simulink model "offGrid_Inverter"  (R2022b)
settings: Solver=FixedStepDiscrete  StartTime=0.0  StopTime=2  FixedStep=1e-6  RelTol=1e-3
libraries: spsSeriesRLCBranchLib x11, spsCurrentMeasurementLib x7, spsMosfetLib x6, slpidlib x5, spsRMSLib x4, simulink x4, spsFourierLib x2, spsTriangleGeneratorLib x2, spsVoltageMeasurementLib x2, spsBreakerLib x1, spsDCVoltageSourceLib x1, spspowerguiLib x1
(part 1 of 2)
settings Model: Creator=XIAO  LastModifiedBy=XIAO
settings SolverCC: AutoInsertRateTranBlk=on
settings DataIOCC: ReturnWorkspaceOutputs=off

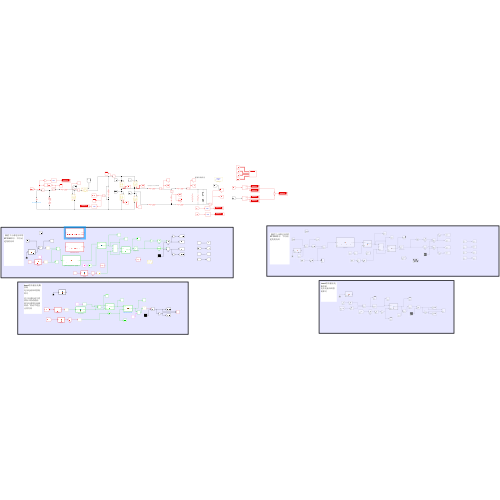
[thumbnail: Simulink's stored preview of the top-level diagram]
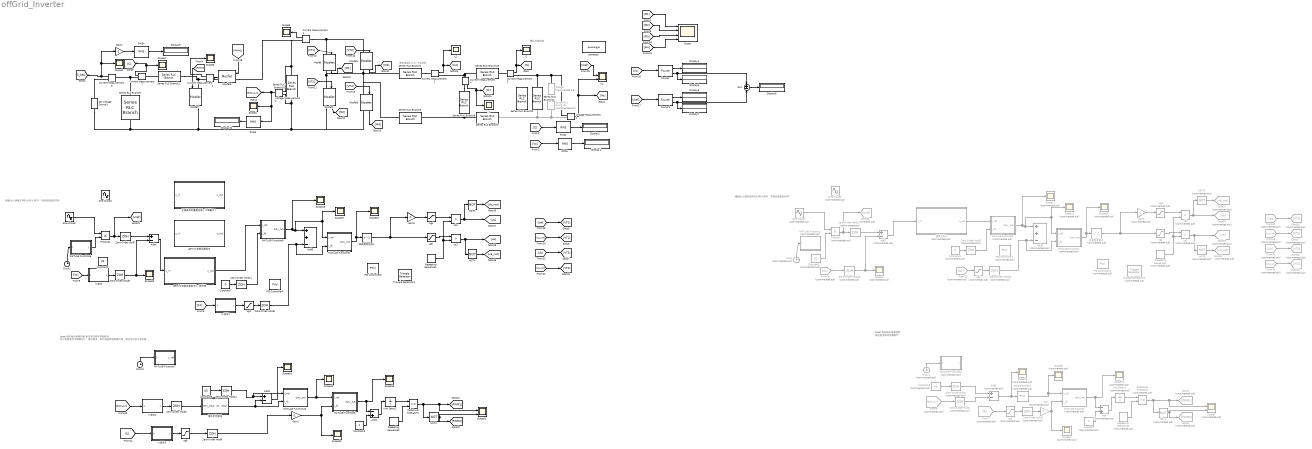
== system offGrid_Inverter ==
  note: boost恒压输出电路控制
      | 电压电流双环控制即可
  note: 模拟负载突变
  note: 寄生电阻大小为：R=2πfL
  note: 幅值大小调电压环的KP和KI即可，不用动逆变的内环
  note: boost恒压输出电路控制
      | 电压电流双环控制即可
      |
      | 对于电感电流不需要加入滑动滤波，因为电感带有高频纹波，滑动平均会让其失真
  note: 幅值大小调电压环的KP和KI即可，不用动逆变的内环
  -ug1 : Saturate  UpperLimit=1  LowerLimit=-1
  -ug2 : Saturate  Commented=on  UpperLimit=1  LowerLimit=-1
  Add : Sum  Commented=on  Inputs=-+
  Add1 : Sum  Inputs=-+
  Add2 : Sum  Commented=on  Inputs=+-
  Add3 : Sum  Inputs=+-
  Add4 : Sum  Inputs=+-
  Add5 : Sum  Inputs=++-
  Add7 : Sum  Commented=on  Inputs=+-
  Add8 : Sum  Commented=on  Inputs=++-
  Breaker : spsBreakerLib/Breaker  Commented=on  InitialState=0  SwitchingTimes=0.6  External=off  BreakerResistance=0.01  SnubberResistance=1e9  SnubberCapacitance=0  Measurements=None  MoreParameters=on  NoBreakLoop=off
  Clock : Clock  Commented=on
  Clock1 : Clock  Commented=on
  Clock2 : Clock
  Clock3 : Clock
  Constant : Constant  Commented=on
  Constant1 : Constant  Commented=on  Value=32
  Constant2 : Constant  Commented=on  Value=55
  Constant3 : Constant  Commented=on  Value=0
  Constant4 : Constant
  Constant5 : Constant  Value=32
  Constant6 : Constant  Value=55
  Constant7 : Constant  Value=0
  Current Measurement{1..7} (7 alike) : spsCurrentMeasurementLib/Current Measurement  PhasorSimulation=off  OutputType=Complex  PSBequivalent=0
  DC Voltage Source1 : spsDCVoltageSourceLib/DC Voltage Source  Amplitude=24  Measurements=None
  Display{1..2,4..10} (9 alike) : Display
  Fourier : spsFourierLib/Fourier  Freq=50  n=1  InInit=[0, 0]  Ts=1e-6
  Fourier1 : spsFourierLib/Fourier  Freq=50  n=1  InInit=[0, 0]  Ts=1e-6
  From28 : From  Commented=on  GotoTag=IL1
  From29 : From  Commented=on  GotoTag=Vo
  From30 : From  Commented=on  GotoTag=ua
  From33 : From  Commented=on  GotoTag=ua_not
  From34 : From  Commented=on  GotoTag=ub_not
  From35 : From  Commented=on  GotoTag=ub
  From5 : From  Commented=on  GotoTag=BUCK_out
  From7 : From  Commented=on  GotoTag=IL
  Gain : Gain  Commented=on  Gain=-1
  Gain1 : Gain  Gain=-1
  Gain2 : Gain  Gain=-1
  Gain3 : Gain  Commented=on  Gain=-1
  Gain4 : Gain  Gain=-1
  Goto26 : Goto  Commented=on  GotoTag=VT1
  Goto27 : Goto  Commented=on  GotoTag=VT2
  Goto28 : Goto  Commented=on  GotoTag=VT3
  Goto29 : Goto  Commented=on  GotoTag=VT4
  Goto30 : Goto  Commented=on  GotoTag=Uref
  Goto31 : Goto  Commented=on  GotoTag=ub_not
  Goto32 : Goto  Commented=on  GotoTag=ub
  Goto33 : Goto  Commented=on  GotoTag=ua
  Goto34 : Goto  Commented=on  GotoTag=ua_not
  Goto8 : Goto  Commented=on  GotoTag=PWM2
  Goto9 : Goto  Commented=on  GotoTag=PWM1
  MATLAB Function : MATLAB Function  Commented=on  TreatAsAtomicUnit=on
  MATLAB Function1 : MATLAB Function  Commented=on  TreatAsAtomicUnit=on
  MATLAB Function10 : MATLAB Function  TreatAsAtomicUnit=on
  MATLAB Function2 : MATLAB Function  Commented=on  TreatAsAtomicUnit=on
  MATLAB Function3 : MATLAB Function  Commented=on  TreatAsAtomicUnit=on
  MATLAB Function4 : MATLAB Function  Commented=on  TreatAsAtomicUnit=on
  MATLAB Function5 : MATLAB Function  TreatAsAtomicUnit=on
  MATLAB Function6 : MATLAB Function  TreatAsAtomicUnit=on
  MATLAB Function7 : MATLAB Function  TreatAsAtomicUnit=on
  MATLAB Function8 : MATLAB Function  TreatAsAtomicUnit=on
  MATLAB Function9 : MATLAB Function  TreatAsAtomicUnit=on
  Mosfet{,1,4..7} (6 alike) : spsMosfetLib/Mosfet  Ron=0.1  Lon=0  Rd=0.01  Vfd=0  IC=0  Rs=1e5  Cs=inf  Measurements=on
  NOT1 : Logic  Commented=on  Operator=NOT  IconShape=distinctive  AllPortsSameDT=off  OutDataTypeStr=boolean
  NOT2 : Logic  Operator=NOT  IconShape=distinctive  AllPortsSameDT=off  OutDataTypeStr=boolean
  NOT3 : Logic  Operator=NOT  IconShape=distinctive  AllPortsSameDT=off  OutDataTypeStr=boolean
  NOT4 : Logic  Operator=NOT  IconShape=distinctive  AllPortsSameDT=off  OutDataTypeStr=boolean
  NOT5 : Logic  Commented=on  Operator=NOT  IconShape=distinctive  AllPortsSameDT=off  OutDataTypeStr=boolean
  NOT6 : Logic  Commented=on  Operator=NOT  IconShape=distinctive  AllPortsSameDT=off  OutDataTypeStr=boolean
  PID Controller1 : slpidlib/PID Controller  Commented=on  Controller=PI  Form=Parallel  TimeDomain=Discrete-time  UseExternalTs=off  SampleTime=-1  IntegratorMethod=Forward Euler  FilterMethod=Forward Euler  ControllerParametersSource=internal  P=0.05  I=4000  UseKiTs=off  D=0  N=100  UseFilter=on  TunerSelectOption=Transfer Function Based (PID Tuner App)  InitialConditionSource=internal  InitialConditionForIntegrator=0  InitialConditionForFilter=0  DifferentiatorICPrevScaledInput=0  ExternalReset=none  TrackingMode=off  Kt=1  LimitOutput=off  SatLimitsSource=internal  UpperSaturationLimit=inf  LowerSaturationLimit=-inf  LinearizeAsGain=on  AntiWindupMode=none  Kb=1  LimitIntegrator=off  UpperIntegratorSaturationLimit=inf  LowerIntegratorSaturationLimit=-inf  POutMin=[]  POutMax=[]  IOutMin=[]  IOutMax=[]  DOutMin=[]  DOutMax=[]  NOutMin=[]  NOutMax=[]  SumOutMin=[]  SumOutMax=[]  SaturationOutMin=[]  SaturationOutMax=[]  PParamMin=[]  PParamMax=[]  IParamMin=[]  IParamMax=[]  DParamMin=[]  DParamMax=[]  NParamMin=[]  NParamMax=[]  KbParamMin=[]  KbParamMax=[]  KtParamMin=[]  KtParamMax=[]  KbOutMin=[]  KbOutMax=[]  KtOutMin=[]  KtOutMax=[]  IntegratorOutMin=[]  IntegratorOutMax=[]  FilterOutMin=[]  FilterOutMax=[]  SumI1OutMin=[]  SumI1OutMax=[]  SumI2OutMin=[]  SumI2OutMax=[]  SumI3OutMin=[]  SumI3OutMax=[]  SumI4OutMin=[]  SumI4OutMax=[]  SumDOutMin=[]  SumDOutMax=[]  DifferentiatorOutMin=[]  DifferentiatorOutMax=[]  FilterDiffOutCoefMin=[]  FilterDiffOutCoefMax=[]  ReciprocalOutMin=[]  ReciprocalOutMax=[]  SumDenOutMin=[]  SumDenOutMax=[]  SumNumOutMin=[]  SumNumOutMax=[]  DivideOutMin=[]  DivideOutMax=[]  UdiffTsProdOutMin=[]  UdiffTsProdOutMax=[]  NTsProdOutMin=[]  NTsProdOutMax=[]  UintegralTsProdOutMin=[]  UintegralTsProdOutMax=[]  UngainTsProdOutMin=[]  UngainTsProdOutMax=[]  ClampingZeroOutDataTypeStr=Inherit: Inherit via back propagation  ClampingZeroOutMin=[]  ClampingZeroOutMax=[]  FilterDenConstantOutDataTypeStr=Inherit: Inherit via back propagation  FilterDenConstantOutMin=[]  FilterDenConstantOutMax=[]  PCopyOutDataTypeStr=Inherit: Inherit via back propagation  PCopyOutMin=[]  PCopyOutMax=[]  NCopyOutDataTypeStr=Inherit: Inherit via back propagation  NCopyOutMin=[]  NCopyOutMax=[]  IntegratorContinuousStateAttributes=''  IntegratorStateMustResolveToSignalObject=off  IntegratorRTWStateStorageClass=Auto  FilterContinuousStateAttributes=''  FilterStateMustResolveToSignalObject=off  FilterRTWStateStorageClass=Auto  ParallelPVariant=InternalParameters  IdealPVariant=Disabled  IVariant=InternalParameters  DVariant=Disabled  IntegratorVariant=Discrete  SatVariant=Disabled  AWVariant=Passthrough  PCopyVariant=Disabled  TRVariant=Disabled  FdbkBlocksVariant=Forward  IdealPFdbkVariant=Disabled  SatFdbkVariant=Disabled  DerivativeFilterVariant=Disabled  NVariant=Disabled  NCopyVariant=Disabled_SignalSpec  FilterICVariant=Disabled  IntegratorICVariant=InternalICs  ExternalResetVariant=Disabled  TRSumVariant=Passthrough  SumFdbkVariant=Disabled  SumVariant=Sum_PI  TsampFilterVariant=InternalTs  TsampNgainVariant=Passthrough  TsampIntegralVariant=Passthrough  ExternalSaturationOutDataTypeStr=Inherit: Same as second input
  PID Controller2 : slpidlib/PID Controller  Commented=on  Controller=PI  Form=Parallel  TimeDomain=Discrete-time  UseExternalTs=off  SampleTime=-1  IntegratorMethod=Forward Euler  FilterMethod=Forward Euler  ControllerParametersSource=internal  P=0.5  I=10  UseKiTs=off  D=0  N=100  UseFilter=on  TunerSelectOption=Transfer Function Based (PID Tuner App)  InitialConditionSource=internal  InitialConditionForIntegrator=0  InitialConditionForFilter=0  DifferentiatorICPrevScaledInput=0  ExternalReset=none  TrackingMode=off  Kt=1  LimitOutput=off  SatLimitsSource=internal  UpperSaturationLimit=inf  LowerSaturationLimit=-inf  LinearizeAsGain=on  AntiWindupMode=none  Kb=1  LimitIntegrator=off  UpperIntegratorSaturationLimit=inf  LowerIntegratorSaturationLimit=-inf  POutMin=[]  POutMax=[]  IOutMin=[]  IOutMax=[]  DOutMin=[]  DOutMax=[]  NOutMin=[]  NOutMax=[]  SumOutMin=[]  SumOutMax=[]  SaturationOutMin=[]  SaturationOutMax=[]  PParamMin=[]  PParamMax=[]  IParamMin=[]  IParamMax=[]  DParamMin=[]  DParamMax=[]  NParamMin=[]  NParamMax=[]  KbParamMin=[]  KbParamMax=[]  KtParamMin=[]  KtParamMax=[]  KbOutMin=[]  KbOutMax=[]  KtOutMin=[]  KtOutMax=[]  IntegratorOutMin=[]  IntegratorOutMax=[]  FilterOutMin=[]  FilterOutMax=[]  SumI1OutMin=[]  SumI1OutMax=[]  SumI2OutMin=[]  SumI2OutMax=[]  SumI3OutMin=[]  SumI3OutMax=[]  SumI4OutMin=[]  SumI4OutMax=[]  SumDOutMin=[]  SumDOutMax=[]  DifferentiatorOutMin=[]  DifferentiatorOutMax=[]  FilterDiffOutCoefMin=[]  FilterDiffOutCoefMax=[]  ReciprocalOutMin=[]  ReciprocalOutMax=[]  SumDenOutMin=[]  SumDenOutMax=[]  SumNumOutMin=[]  SumNumOutMax=[]  DivideOutMin=[]  DivideOutMax=[]  UdiffTsProdOutMin=[]  UdiffTsProdOutMax=[]  NTsProdOutMin=[]  NTsProdOutMax=[]  UintegralTsProdOutMin=[]  UintegralTsProdOutMax=[]  UngainTsProdOutMin=[]  UngainTsProdOutMax=[]  ClampingZeroOutDataTypeStr=Inherit: Inherit via back propagation  ClampingZeroOutMin=[]  ClampingZeroOutMax=[]  FilterDenConstantOutDataTypeStr=Inherit: Inherit via back propagation  FilterDenConstantOutMin=[]  FilterDenConstantOutMax=[]  PCopyOutDataTypeStr=Inherit: Inherit via back propagation  PCopyOutMin=[]  PCopyOutMax=[]  NCopyOutDataTypeStr=Inherit: Inherit via back propagation  NCopyOutMin=[]  NCopyOutMax=[]  IntegratorContinuousStateAttributes=''  IntegratorStateMustResolveToSignalObject=off  IntegratorRTWStateStorageClass=Auto  FilterContinuousStateAttributes=''  FilterStateMustResolveToSignalObject=off  FilterRTWStateStorageClass=Auto  ParallelPVariant=InternalParameters  IdealPVariant=Disabled  IVariant=InternalParameters  DVariant=Disabled  IntegratorVariant=Discrete  SatVariant=Disabled  AWVariant=Passthrough  PCopyVariant=Disabled  TRVariant=Disabled  FdbkBlocksVariant=Forward  IdealPFdbkVariant=Disabled  SatFdbkVariant=Disabled  DerivativeFilterVariant=Disabled  NVariant=Disabled  NCopyVariant=Disabled_SignalSpec  FilterICVariant=Disabled  IntegratorICVariant=InternalICs  ExternalResetVariant=Disabled  TRSumVariant=Passthrough  SumFdbkVariant=Disabled  SumVariant=Sum_PI  TsampFilterVariant=InternalTs  TsampNgainVariant=Passthrough  TsampIntegralVariant=Passthrough  ExternalSaturationOutDataTypeStr=Inherit: Same as second input
  PID Controller3 : slpidlib/PID Controller  Commented=on  Controller=PI  Form=Parallel  TimeDomain=Discrete-time  UseExternalTs=off  SampleTime=-1  IntegratorMethod=Forward Euler  FilterMethod=Forward Euler  ControllerParametersSource=internal  P=0.1  I=0  UseKiTs=off  D=0  N=100  UseFilter=on  TunerSelectOption=Transfer Function Based (PID Tuner App)  InitialConditionSource=internal  InitialConditionForIntegrator=0  InitialConditionForFilter=0  DifferentiatorICPrevScaledInput=0  ExternalReset=none  TrackingMode=off  Kt=1  LimitOutput=off  SatLimitsSource=internal  UpperSaturationLimit=inf  LowerSaturationLimit=-inf  LinearizeAsGain=on  AntiWindupMode=none  Kb=1  LimitIntegrator=off  UpperIntegratorSaturationLimit=inf  LowerIntegratorSaturationLimit=-inf  POutMin=[]  POutMax=[]  IOutMin=[]  IOutMax=[]  DOutMin=[]  DOutMax=[]  NOutMin=[]  NOutMax=[]  SumOutMin=[]  SumOutMax=[]  SaturationOutMin=[]  SaturationOutMax=[]  PParamMin=[]  PParamMax=[]  IParamMin=[]  IParamMax=[]  DParamMin=[]  DParamMax=[]  NParamMin=[]  NParamMax=[]  KbParamMin=[]  KbParamMax=[]  KtParamMin=[]  KtParamMax=[]  KbOutMin=[]  KbOutMax=[]  KtOutMin=[]  KtOutMax=[]  IntegratorOutMin=[]  IntegratorOutMax=[]  FilterOutMin=[]  FilterOutMax=[]  SumI1OutMin=[]  SumI1OutMax=[]  SumI2OutMin=[]  SumI2OutMax=[]  SumI3OutMin=[]  SumI3OutMax=[]  SumI4OutMin=[]  SumI4OutMax=[]  SumDOutMin=[]  SumDOutMax=[]  DifferentiatorOutMin=[]  DifferentiatorOutMax=[]  FilterDiffOutCoefMin=[]  FilterDiffOutCoefMax=[]  ReciprocalOutMin=[]  ReciprocalOutMax=[]  SumDenOutMin=[]  SumDenOutMax=[]  SumNumOutMin=[]  SumNumOutMax=[]  DivideOutMin=[]  DivideOutMax=[]  UdiffTsProdOutMin=[]  UdiffTsProdOutMax=[]  NTsProdOutMin=[]  NTsProdOutMax=[]  UintegralTsProdOutMin=[]  UintegralTsProdOutMax=[]  UngainTsProdOutMin=[]  UngainTsProdOutMax=[]  ClampingZeroOutDataTypeStr=Inherit: Inherit via back propagation  ClampingZeroOutMin=[]  ClampingZeroOutMax=[]  FilterDenConstantOutDataTypeStr=Inherit: Inherit via back propagation  FilterDenConstantOutMin=[]  FilterDenConstantOutMax=[]  PCopyOutDataTypeStr=Inherit: Inherit via back propagation  PCopyOutMin=[]  PCopyOutMax=[]  NCopyOutDataTypeStr=Inherit: Inherit via back propagation  NCopyOutMin=[]  NCopyOutMax=[]  IntegratorContinuousStateAttributes=''  IntegratorStateMustResolveToSignalObject=off  IntegratorRTWStateStorageClass=Auto  FilterContinuousStateAttributes=''  FilterStateMustResolveToSignalObject=off  FilterRTWStateStorageClass=Auto  ParallelPVariant=InternalParameters  IdealPVariant=Disabled  IVariant=InternalParameters  DVariant=Disabled  IntegratorVariant=Discrete  SatVariant=Disabled  AWVariant=Passthrough  PCopyVariant=Disabled  TRVariant=Disabled  FdbkBlocksVariant=Forward  IdealPFdbkVariant=Disabled  SatFdbkVariant=Disabled  DerivativeFilterVariant=Disabled  NVariant=Disabled  NCopyVariant=Disabled_SignalSpec  FilterICVariant=Disabled  IntegratorICVariant=InternalICs  ExternalResetVariant=Disabled  TRSumVariant=Passthrough  SumFdbkVariant=Disabled  SumVariant=Sum_PI  TsampFilterVariant=InternalTs  TsampNgainVariant=Passthrough  TsampIntegralVariant=Passthrough  ExternalSaturationOutDataTypeStr=Inherit: Same as second input
  PID Controller4 : slpidlib/PID Controller  Controller=PI  Form=Parallel  TimeDomain=Discrete-time  UseExternalTs=off  SampleTime=-1  IntegratorMethod=Forward Euler  FilterMethod=Forward Euler  ControllerParametersSource=internal  P=0.05  I=4000  UseKiTs=off  D=0  N=100  UseFilter=on  TunerSelectOption=Transfer Function Based (PID Tuner App)  InitialConditionSource=internal  InitialConditionForIntegrator=0  InitialConditionForFilter=0  DifferentiatorICPrevScaledInput=0  ExternalReset=none  TrackingMode=off  Kt=1  LimitOutput=off  SatLimitsSource=internal  UpperSaturationLimit=inf  LowerSaturationLimit=-inf  LinearizeAsGain=on  AntiWindupMode=none  Kb=1  LimitIntegrator=off  UpperIntegratorSaturationLimit=inf  LowerIntegratorSaturationLimit=-inf  POutMin=[]  POutMax=[]  IOutMin=[]  IOutMax=[]  DOutMin=[]  DOutMax=[]  NOutMin=[]  NOutMax=[]  SumOutMin=[]  SumOutMax=[]  SaturationOutMin=[]  SaturationOutMax=[]  PParamMin=[]  PParamMax=[]  IParamMin=[]  IParamMax=[]  DParamMin=[]  DParamMax=[]  NParamMin=[]  NParamMax=[]  KbParamMin=[]  KbParamMax=[]  KtParamMin=[]  KtParamMax=[]  KbOutMin=[]  KbOutMax=[]  KtOutMin=[]  KtOutMax=[]  IntegratorOutMin=[]  IntegratorOutMax=[]  FilterOutMin=[]  FilterOutMax=[]  SumI1OutMin=[]  SumI1OutMax=[]  SumI2OutMin=[]  SumI2OutMax=[]  SumI3OutMin=[]  SumI3OutMax=[]  SumI4OutMin=[]  SumI4OutMax=[]  SumDOutMin=[]  SumDOutMax=[]  DifferentiatorOutMin=[]  DifferentiatorOutMax=[]  FilterDiffOutCoefMin=[]  FilterDiffOutCoefMax=[]  ReciprocalOutMin=[]  ReciprocalOutMax=[]  SumDenOutMin=[]  SumDenOutMax=[]  SumNumOutMin=[]  SumNumOutMax=[]  DivideOutMin=[]  DivideOutMax=[]  UdiffTsProdOutMin=[]  UdiffTsProdOutMax=[]  NTsProdOutMin=[]  NTsProdOutMax=[]  UintegralTsProdOutMin=[]  UintegralTsProdOutMax=[]  UngainTsProdOutMin=[]  UngainTsProdOutMax=[]  ClampingZeroOutDataTypeStr=Inherit: Inherit via back propagation  ClampingZeroOutMin=[]  ClampingZeroOutMax=[]  FilterDenConstantOutDataTypeStr=Inherit: Inherit via back propagation  FilterDenConstantOutMin=[]  FilterDenConstantOutMax=[]  PCopyOutDataTypeStr=Inherit: Inherit via back propagation  PCopyOutMin=[]  PCopyOutMax=[]  NCopyOutDataTypeStr=Inherit: Inherit via back propagation  NCopyOutMin=[]  NCopyOutMax=[]  IntegratorContinuousStateAttributes=''  IntegratorStateMustResolveToSignalObject=off  IntegratorRTWStateStorageClass=Auto  FilterContinuousStateAttributes=''  FilterStateMustResolveToSignalObject=off  FilterRTWStateStorageClass=Auto  ParallelPVariant=InternalParameters  IdealPVariant=Disabled  IVariant=InternalParameters  DVariant=Disabled  IntegratorVariant=Discrete  SatVariant=Disabled  AWVariant=Passthrough  PCopyVariant=Disabled  TRVariant=Disabled  FdbkBlocksVariant=Forward  IdealPFdbkVariant=Disabled  SatFdbkVariant=Disabled  DerivativeFilterVariant=Disabled  NVariant=Disabled  NCopyVariant=Disabled_SignalSpec  FilterICVariant=Disabled  IntegratorICVariant=InternalICs  ExternalResetVariant=Disabled  TRSumVariant=Passthrough  SumFdbkVariant=Disabled  SumVariant=Sum_PI  TsampFilterVariant=InternalTs  TsampNgainVariant=Passthrough  TsampIntegralVariant=Passthrough  ExternalSaturationOutDataTypeStr=Inherit: Same as second input
  PID Controller6 : slpidlib/PID Controller  Controller=PI  Form=Parallel  TimeDomain=Discrete-time  UseExternalTs=off  SampleTime=-1  IntegratorMethod=Forward Euler  FilterMethod=Forward Euler  ControllerParametersSource=internal  P=0.1  I=0  UseKiTs=off  D=0  N=100  UseFilter=on  TunerSelectOption=Transfer Function Based (PID Tuner App)  InitialConditionSource=internal  InitialConditionForIntegrator=0  InitialConditionForFilter=0  DifferentiatorICPrevScaledInput=0  ExternalReset=none  TrackingMode=off  Kt=1  LimitOutput=off  SatLimitsSource=internal  UpperSaturationLimit=inf  LowerSaturationLimit=-inf  LinearizeAsGain=on  AntiWindupMode=none  Kb=1  LimitIntegrator=off  UpperIntegratorSaturationLimit=inf  LowerIntegratorSaturationLimit=-inf  POutMin=[]  POutMax=[]  IOutMin=[]  IOutMax=[]  DOutMin=[]  DOutMax=[]  NOutMin=[]  NOutMax=[]  SumOutMin=[]  SumOutMax=[]  SaturationOutMin=[]  SaturationOutMax=[]  PParamMin=[]  PParamMax=[]  IParamMin=[]  IParamMax=[]  DParamMin=[]  DParamMax=[]  NParamMin=[]  NParamMax=[]  KbParamMin=[]  KbParamMax=[]  KtParamMin=[]  KtParamMax=[]  KbOutMin=[]  KbOutMax=[]  KtOutMin=[]  KtOutMax=[]  IntegratorOutMin=[]  IntegratorOutMax=[]  FilterOutMin=[]  FilterOutMax=[]  SumI1OutMin=[]  SumI1OutMax=[]  SumI2OutMin=[]  SumI2OutMax=[]  SumI3OutMin=[]  SumI3OutMax=[]  SumI4OutMin=[]  SumI4OutMax=[]  SumDOutMin=[]  SumDOutMax=[]  DifferentiatorOutMin=[]  DifferentiatorOutMax=[]  FilterDiffOutCoefMin=[]  FilterDiffOutCoefMax=[]  ReciprocalOutMin=[]  ReciprocalOutMax=[]  SumDenOutMin=[]  SumDenOutMax=[]  SumNumOutMin=[]  SumNumOutMax=[]  DivideOutMin=[]  DivideOutMax=[]  UdiffTsProdOutMin=[]  UdiffTsProdOutMax=[]  NTsProdOutMin=[]  NTsProdOutMax=[]  UintegralTsProdOutMin=[]  UintegralTsProdOutMax=[]  UngainTsProdOutMin=[]  UngainTsProdOutMax=[]  ClampingZeroOutDataTypeStr=Inherit: Inherit via back propagation  ClampingZeroOutMin=[]  ClampingZeroOutMax=[]  FilterDenConstantOutDataTypeStr=Inherit: Inherit via back propagation  FilterDenConstantOutMin=[]  FilterDenConstantOutMax=[]  PCopyOutDataTypeStr=Inherit: Inherit via back propagation  PCopyOutMin=[]  PCopyOutMax=[]  NCopyOutDataTypeStr=Inherit: Inherit via back propagation  NCopyOutMin=[]  NCopyOutMax=[]  IntegratorContinuousStateAttributes=''  IntegratorStateMustResolveToSignalObject=off  IntegratorRTWStateStorageClass=Auto  FilterContinuousStateAttributes=''  FilterStateMustResolveToSignalObject=off  FilterRTWStateStorageClass=Auto  ParallelPVariant=InternalParameters  IdealPVariant=Disabled  IVariant=InternalParameters  DVariant=Disabled  IntegratorVariant=Discrete  SatVariant=Disabled  AWVariant=Passthrough  PCopyVariant=Disabled  TRVariant=Disabled  FdbkBlocksVariant=Forward  IdealPFdbkVariant=Disabled  SatFdbkVariant=Disabled  DerivativeFilterVariant=Disabled  NVariant=Disabled  NCopyVariant=Disabled_SignalSpec  FilterICVariant=Disabled  IntegratorICVariant=InternalICs  ExternalResetVariant=Disabled  TRSumVariant=Passthrough  SumFdbkVariant=Disabled  SumVariant=Sum_PI  TsampFilterVariant=InternalTs  TsampNgainVariant=Passthrough  TsampIntegralVariant=Passthrough  ExternalSaturationOutDataTypeStr=Inherit: Same as second input
  Product : Product  Commented=on
  Product1 : Product
  RMS1 : spsRMSLib/RMS  TrueRMS=on  Freq=50  RMSInit=24  Ts=1e-6
  RMS2 : spsRMSLib/RMS  TrueRMS=on  Freq=50  RMSInit=24  Ts=1e-6
  RMS4 : spsRMSLib/RMS  TrueRMS=on  Freq=50  RMSInit=120  Ts=1e-6
  RMS5 : spsRMSLib/RMS  TrueRMS=on  Freq=50  RMSInit=120  Ts=1e-6
  Relational Operator1 : RelationalOperator  Commented=on  OutDataTypeStr=boolean  RndMeth=Simplest  InputSameDT=off
  Relational Operator2 : RelationalOperator  OutDataTypeStr=boolean  RndMeth=Simplest  InputSameDT=off
  Repeating Sequence1 : simulink/Sources/Repeating Sequence  Commented=on  rep_seq_t=[0 0.00005 0.0001]  rep_seq_y=[0 1 0]
  Repeating Sequence2 : simulink/Sources/Repeating Sequence  Commented=on  rep_seq_t=[0 0.00005 0.0001]  rep_seq_y=[-1 1 -1]
  Repeating Sequence3 : simulink/Sources/Repeating Sequence  rep_seq_t=[0 0.00005 0.0001]  rep_seq_y=[0 1 0]
  Repeating Sequence4 : simulink/Sources/Repeating Sequence  rep_seq_t=[0 0.00005 0.0001]  rep_seq_y=[-1 1 -1]
  Scope : Scope  NumInputPorts=4
  Scope{1..3,5..6,15..20,22..23} (13 alike) : Scope
  Scope{4,8..14} (8 alike) : Scope  Commented=on
  Scope21 : Scope  NumInputPorts=2
  Scope7 : Scope  Commented=on  NumInputPorts=2
  Series RLC Branch1 : spsSeriesRLCBranchLib/Series RLC Branch  LConnTagsString=__new0  RConnTagsString=__new0  BranchType=RL  Resistance=0.1  Inductance=2.5e-3  SetiL0=off  InitialCurrent=0  Capacitance=1e-6  Setx0=off  InitialVoltage=0  Measurements=None
  Series RLC Branch10 : spsSeriesRLCBranchLib/Series RLC Branch  LConnTagsString=__new0  RConnTagsString=__new0  BranchType=RC  Resistance=0.01  Inductance=0  SetiL0=off  InitialCurrent=0  Capacitance=1880e-6  Setx0=off  InitialVoltage=0  Measurements=None
  Series RLC Branch11 : spsSeriesRLCBranchLib/Series RLC Branch  Commented=on  LConnTagsString=__new0  RConnTagsString=__new0  BranchType=R  Resistance=16  Inductance=0  SetiL0=off  InitialCurrent=0  Capacitance=22e-6  Setx0=off  InitialVoltage=0  Measurements=None
  Series RLC Branch12 : spsSeriesRLCBranchLib/Series RLC Branch  LConnTagsString=__new0  RConnTagsString=__new0  BranchType=R  Resistance=16  Inductance=10e-3  SetiL0=off  InitialCurrent=0  Capacitance=220e-6  Setx0=off  InitialVoltage=0  Measurements=None
  Series RLC Branch13 : spsSeriesRLCBranchLib/Series RLC Branch  LConnTagsString=__new0  RConnTagsString=__new0  BranchType=RL  Resistance=0.1  Inductance=0.00012  SetiL0=off  InitialCurrent=0  Capacitance=220e-6  Setx0=off  InitialVoltage=0  Measurements=None
  Series RLC Branch2 : spsSeriesRLCBranchLib/Series RLC Branch  LConnTagsString=__new0  RConnTagsString=__new0  BranchType=RL  Resistance=0.1  Inductance=0.0015  SetiL0=off  InitialCurrent=0  Capacitance=220e-6  Setx0=off  InitialVoltage=0  Measurements=None
  Series RLC Branch3 : spsSeriesRLCBranchLib/Series RLC Branch  LConnTagsString=__new0  RConnTagsString=__new0  BranchType=RL  Resistance=0.1  Inductance=0.0015  SetiL0=off  InitialCurrent=0  Capacitance=220e-6  Setx0=off  InitialVoltage=0  Measurements=None
  Series RLC Branch4 : spsSeriesRLCBranchLib/Series RLC Branch  LConnTagsString=__new0  RConnTagsString=__new0  BranchType=RL  Resistance=0.1  Inductance=0.00012  SetiL0=off  InitialCurrent=0  Capacitance=220e-6  Setx0=off  InitialVoltage=0  Measurements=None
  Series RLC Branch7 : spsSeriesRLCBranchLib/Series RLC Branch  LConnTagsString=__new0  RConnTagsString=__new0  BranchType=RC  Resistance=0.1  Inductance=1e-3  SetiL0=off  InitialCurrent=0  Capacitance=940e-6  Setx0=off  InitialVoltage=0  Measurements=None
  Series RLC Branch8 : spsSeriesRLCBranchLib/Series RLC Branch  LConnTagsString=__new0  RConnTagsString=__new0  BranchType=RC  Resistance=0.01  Inductance=0  SetiL0=off  InitialCurrent=0  Capacitance=10e-6  Setx0=off  InitialVoltage=0  Measurements=None
  Series RLC Branch9 : spsSeriesRLCBranchLib/Series RLC Branch  LConnTagsString=__new0  RConnTagsString=__new0  BranchType=R  Resistance=1e9  Inductance=0.01  SetiL0=off  InitialCurrent=0  Capacitance=22e-6  Setx0=off  InitialVoltage=0  Measurements=None
  Sine Wave1 : Sin  Commented=on  Amplitude=1*1.414  Frequency=100*pi  SampleTime=0
  Sine Wave2 : Sin  Amplitude=1*1.414  Frequency=100*pi  SampleTime=0
  Sine Wave3 : Sin  Commented=on  Amplitude=32*1.414  Frequency=100*pi  SampleTime=0
  Sine Wave4 : Sin  Amplitude=32*1.414  Frequency=100*pi  SampleTime=0
  Sum : Sum  Inputs=+-
  Triangle Generator1 : spsTriangleGeneratorLib/Triangle Generator  Freq=10000  Phase=90  Ts=0
  Triangle Generator3 : spsTriangleGeneratorLib/Triangle Generator  Commented=on  Freq=10000  Phase=90  Ts=0
  Unit Delay1 : UnitDelay  Commented=on  SampleTime=5e-5  HasFrameUpgradeWarning=on
  Unit Delay2 : UnitDelay  SampleTime=5e-5  HasFrameUpgradeWarning=on
  Vo : Scope  NumInputPorts=2
  Voltage Measurement1 : spsVoltageMeasurementLib/Voltage Measurement  PhasorSimulation=off  OutputType=Complex  PSBequivalent=0
  Voltage Measurement2 : spsVoltageMeasurementLib/Voltage Measurement  PhasorSimulation=off  OutputType=Complex  PSBequivalent=0
  Zero-Order Hold{1..4,10,12..13} (7 alike) : ZeroOrderHold  Commented=on  SampleTime=5e-5
  Zero-Order Hold{5..9,11,14} (7 alike) : ZeroOrderHold  SampleTime=5e-5
  gemini简便运算版本 : MATLAB Function  TreatAsAtomicUnit=on
  gemini简便运算版本1，更快捷 : MATLAB Function  TreatAsAtomicUnit=on
  i1 : Scope
  i2 : Scope
  iL1 : Scope
  powergui : spspowerguiLib/powergui  Priority=1  SimulationMode=Discrete  SampleTime=1e-6  frequency=60  Iterations=50  frequencyindice=0  Pbase=100e6  ErrMax=1e-4  UnitsV=kV  UnitsW=MW  buscounter=0  FunctionMessages=off  echomessages=off  EnableUseOfTLC=off  CurrentSourceSwitches=off  DisableSnubberDevices=off  DisableRonSwitches=off  DisableVfSwitches=off  DisplayEquations=off  AutomaticDiscreteSolvers=off  SolverType=Tustin/Backward Euler (TBE)  Interpol=off  ExternalGateDelay=off  methode=off  Ts=100  x0status=blocks  SPID=on  SwTol=0  HookPort=off  NonlinearTolerance=1e-4  nMaxIteration=100  ContinueOnMaxIteration=off  RestoreLinks=warning  ResistiveCurrentMeasurement=off  Frange=[0:2:500]  Ylog=off  Xlog=on  ShowGrid=off  save=off  variable=ZData  structure=0  ZoomFFT=off  StartTime=0.0  cycles=1  DisplayStyle=1  fundamental=60  FreqAxis=off  MaxFrequency=1000  frequencyindicesteady=1  RmsSteady=1  display=off
  rc滤波 : MATLAB Function  TreatAsAtomicUnit=on
  rc滤波1 : MATLAB Function  TreatAsAtomicUnit=on
  rc滤波2 : MATLAB Function  TreatAsAtomicUnit=on
  rc滤波3 : MATLAB Function  TreatAsAtomicUnit=on
  ua1 : RelationalOperator  Operator=>  OutDataTypeStr=boolean  RndMeth=Simplest  InputSameDT=off
  ua2 : RelationalOperator  Commented=on  Operator=>  OutDataTypeStr=boolean  RndMeth=Simplest  InputSameDT=off
  ub1 : RelationalOperator  Operator=>  OutDataTypeStr=boolean  RndMeth=Simplest  InputSameDT=off
  ub2 : RelationalOperator  Commented=on  Operator=>  OutDataTypeStr=boolean  RndMeth=Simplest  InputSameDT=off
  ug1 : Saturate  Commented=on  UpperLimit=5  LowerLimit=-5
  ug2 : Saturate  Commented=on  UpperLimit=1  LowerLimit=-1
  ug3 : Saturate  Commented=on  UpperLimit=10  LowerLimit=-10
  ug4 : Saturate  UpperLimit=5  LowerLimit=-5
  ug5 : Saturate  UpperLimit=1  LowerLimit=-1
  ug6 : Saturate  UpperLimit=10  LowerLimit=-10
  数据更新延迟 : Delay  Commented=on  DelayLength=1  SampleTime=5e-5
  数据更新延迟1 : Delay  DelayLength=1  SampleTime=5e-5
  正确版本的重复控制（计算量大） : MATLAB Function  TreatAsAtomicUnit=on
  滑动平均滤波 : MATLAB Function  TreatAsAtomicUnit=on
  重复控制1 : MATLAB Function  Commented=on  TreatAsAtomicUnit=on
  wires:
  Unit Delay1/1 -> Relational Operator1/1
  Zero-Order Hold4/1 -> Add2/1
  PID Controller2/1 -> Scope8/1, MATLAB Function/1(I_ref)
  Zero-Order Hold1/1 -> Add2/2
  Relational Operator1/1 -> NOT1/1, Goto9/1, Scope7/1
  NOT1/1 -> Goto8/1, Scope7/2
  Repeating Sequence1/1 -> Relational Operator1/2
  MATLAB Function/1(duty_out) -> Add/1, Scope10/1
  From5/1 -> Zero-Order Hold1/1
  Add2/1 -> Scope13/1, PID Controller2/1
  Gain/1 -> Scope9/1, MATLAB Function/2(I_fb)
  From7/1 -> ug3/1
  ua2/1 -> NOT6/1, Goto33/1
  From33/1 -> Goto27/1
  From35/1 -> Goto28/1
  -ug2/1 -> ub2/1
  [VT4] -> Mosfet5/1
  [Uref] -> Vo/1
  NOT6/1 -> Goto34/1
  Current Measurement5/1 -> i2/1, [I2]
  Zero-Order Hold12/1 -> Add7/1
  Mosfet1/1 -> [M2]
  From29/1 -> Zero-Order Hold10/1
  From30/1 -> Goto26/1
  NOT5/1 -> Goto31/1
  Gain3/1 -> -ug2/1
  [Vo] -> Fourier/1
  Current Measurement4/1 -> i1/1, [IC]
  From34/1 -> Goto29/1
  Fourier/1 -> Display4/1
  [Vo] -> RMS1/1
  [I2] -> RMS2/1
  RMS2/1 -> Display2/1
  Sum/1 -> Display8/1
  Fourier1/2 -> Sum/2, Display7/1
  [M3] -> Scope/3
  Fourier1/1 -> Display6/1
  Fourier/2 -> Display5/1, Sum/1
  [Uref] -> Fourier1/1
  [M4] -> Scope/4
  Current Measurement1/1 -> iL1/1, [IL1]
  [VT1] -> Mosfet/1
  Mosfet/1 -> [M1]
  ug2/1 -> ua2/1
  RMS1/1 -> Display1/1
  [M1] -> Scope/1
  Mosfet5/1 -> [M4]
  ub2/1 -> NOT5/1, Goto32/1
  Voltage Measurement1/1 -> [Vo], Vo/2
  [VT3] -> Mosfet4/1
  [M2] -> Scope/2
  [VT2] -> Mosfet1/1
  Mosfet4/1 -> [M3]
  Zero-Order Hold10/1 -> Add7/2, Scope4/1
  RMS4/1 -> Display9/1
  Gain2/1 -> RMS4/1
  [PWM2] -> Mosfet7/1
  Current Measurement6/1 -> Scope1/1, Gain2/1, [i_bat]
  [PWM1] -> Mosfet6/1
  Voltage Measurement2/1 -> RMS5/1, Scope2/1, [BUCK_out]
  RMS5/1 -> Display10/1
  Current Measurement7/1 -> Scope3/1, [IL]
  Current Measurement2/1 -> Scope5/1
  Current Measurement3/1 -> Scope6/1
  From28/1 -> ug1/1
  Zero-Order Hold13/1 -> MATLAB Function4/2(I_fb), Add8/3
  Zero-Order Hold2/1 -> Gain/1
  ug3/1 -> Zero-Order Hold2/1
  ug1/1 -> Zero-Order Hold13/1
  Add7/1 -> 重复控制1/1(u_in)
  Sine Wave1/1 -> Product/1
  Clock/1 -> MATLAB Function1/1(t)
  Product/1 -> Goto30/1, Zero-Order Hold12/1
  数据更新延迟/1 -> Gain3/1, ug2/1
  Repeating Sequence2/1 -> ub2/2, ua2/2
  Constant/1 -> Add/2
  Add/1 -> Unit Delay1/1
  Constant1/1 -> Product/2
  Constant3/1 -> Zero-Order Hold3/1
  Zero-Order Hold3/1 -> MATLAB Function3/2(I_fb)
  重复控制1/1(u_out) -> MATLAB Function3/1(I_ref)
  MATLAB Function3/1(duty_out) -> MATLAB Function4/1(I_ref), Scope12/1, Add8/1, Scope11/1
  Clock1/1 -> MATLAB Function2/1(t)
  Constant2/1 -> Zero-Order Hold4/1
  MATLAB Function4/1(duty_out) -> Scope14/1, 数据更新延迟/1
  Relational Operator2/1 -> NOT2/1, [PWM1], Scope21/1
  Zero-Order Hold5/1 -> 滑动平均滤波/1(IGm_total)
  Unit Delay2/1 -> Relational Operator2/1
  Repeating Sequence4/1 -> ub1/2, ua1/2
  Gain4/1 -> -ug1/1
  [BUCK_out] -> rc滤波2/1(u)
  -ug1/1 -> ub1/1
  [ua_not] -> [VT2]
  MATLAB Function5/1(duty_out) -> Add1/1, Scope15/1
  Constant4/1 -> Add1/2
  Zero-Order Hold11/1 -> MATLAB Function8/2(I_fb)
  [Vo] -> rc滤波/1(u)
  MATLAB Function9/1(duty_out) -> Scope19/1, 数据更新延迟1/1
  [ua] -> [VT1]
  ug6/1 -> Zero-Order Hold9/1
  MATLAB Function8/1(duty_out) -> MATLAB Function9/1(I_ref), Scope17/1, Add5/1, Scope16/1
  Sine Wave2/1 -> Product1/1
  ua1/1 -> NOT4/1, [ua]
  Zero-Order Hold7/1 -> Add4/1
  [ub] -> [VT3]
  [IL1] -> rc滤波1/1(u)
  数据更新延迟1/1 -> Gain4/1, ug5/1
  Add1/1 -> Unit Delay2/1
  Product1/1 -> [Uref], Zero-Order Hold7/1
  Clock3/1 -> MATLAB Function7/1(t)
  Clock2/1 -> MATLAB Function6/1(t)
  ug4/1 -> Zero-Order Hold8/1
  Add3/1 -> Scope18/1
  ub1/1 -> NOT3/1, [ub]
  NOT4/1 -> [ua_not]
  Gain1/1 -> Scope23/1, MATLAB Function5/2(I_fb)
  [IL] -> rc滤波3/1(u)
  Constant7/1 -> Zero-Order Hold11/1
  [ub_not] -> [VT4]
  Zero-Order Hold14/1 -> MATLAB Function10/1(I_ref), Add3/1
  NOT2/1 -> [PWM2], Scope21/2
  Repeating Sequence3/1 -> Relational Operator2/2
  Zero-Order Hold8/1 -> MATLAB Function9/2(I_fb), Add5/3
  Zero-Order Hold6/1 -> Add4/2, Scope20/1
  ug5/1 -> ua1/1
  NOT3/1 -> [ub_not]
  rc滤波/1(y) -> Zero-Order Hold6/1
  rc滤波1/1(y) -> ug4/1
  rc滤波2/1(y) -> Zero-Order Hold5/1
  rc滤波3/1(y) -> ug6/1
  MATLAB Function10/1(duty_out) -> Scope22/1, MATLAB Function5/1(I_ref)
  滑动平均滤波/1(IGm_clean) -> Add3/2, MATLAB Function10/2(I_fb)
  Zero-Order Hold9/1 -> Gain1/1
  Constant6/1 -> Zero-Order Hold14/1
  MATLAB Function6/1(y) -> Product1/2
  Add4/1 -> gemini简便运算版本1，更快捷/1(u_in)
  gemini简便运算版本1，更快捷/1(u_out) -> MATLAB Function8/1(I_ref)
  connections:
  Mosfet7/RConn1 -- DC Voltage Source1/LConn1 -- Series RLC Branch7/RConn1 -- Mosfet5/RConn1 -- Mosfet1/RConn1 -- Voltage Measurement2/LConn2 -- Series RLC Branch10/RConn1
  Mosfet4/RConn1 -- Series RLC Branch3/RConn1 -- Mosfet5/LConn1
  Voltage Measurement2/LConn1 -- Current Measurement3/RConn1 -- Mosfet6/LConn1 -- Series RLC Branch10/LConn1
  Current Measurement5/RConn1 -- Voltage Measurement1/LConn1 -- Breaker/RConn1 -- Series RLC Branch12/RConn1
  Series RLC Branch2/RConn1 -- Mosfet/RConn1 -- Mosfet1/LConn1
  Current Measurement4/LConn1 -- Current Measurement1/RConn1 -- Series RLC Branch13/RConn1
  Current Measurement5/LConn1 -- Series RLC Branch13/LConn1
  Breaker/LConn1 -- Series RLC Branch11/LConn1
  Series RLC Branch2/LConn1 -- Current Measurement1/LConn1
  Current Measurement4/RConn1 -- Series RLC Branch8/LConn1
  Current Measurement7/RConn1 -- Current Measurement6/LConn1 -- Series RLC Branch7/LConn1
  Series RLC Branch1/LConn1 -- Current Measurement2/RConn1 -- Mosfet7/LConn1
  Series RLC Branch1/RConn1 -- Current Measurement7/LConn1
  Current Measurement6/RConn1 -- DC Voltage Source1/RConn1
  Series RLC Branch8/RConn1 -- Series RLC Branch4/RConn1 -- Series RLC Branch3/LConn1
  Series RLC Branch11/RConn1 -- Series RLC Branch4/LConn1 -- Series RLC Branch12/LConn1 -- Voltage Measurement1/LConn2
  Current Measurement2/LConn1 -- Mosfet6/RConn1
  Mosfet4/LConn1 -- Mosfet/LConn1 -- Current Measurement3/LConn1

== matlab function offGrid_Inverter/rc滤波2 ==
  data: u input; y output
function y = fcn(u)
% 一阶RC低通滤波（数字等效实现）
% 适配：仿真步长 Ts=1e-6s（Fs=1MHz），截止频率 fc=4.7kHz
% 输入：u - 原始信号
% 输出：y - RC滤波后的信号

% persistent 变量保存上一时刻的输出（RC滤波的状态）
persistent y_prev;

% ---------------- 固定参数（已按你的需求预计算） ----------------
fc = 4700;   % 截止频率：4.7kHz
Ts = 1e-6;   % 仿真步长：1us（1e-6s）
tau = 1/(2*pi*fc); % RC时间常数 τ=RC=1/(2πfc)
alpha = exp(-Ts/tau); % 滤波系数（RC离散化核心）
% ----------------------------------------------------------------

% 初始化状态（仅第一次调用时执行，默认初始输出为0）
if isempty(y_prev)
    y_prev = 0;
end

% 一阶RC低通的离散差分方程（和真实RC电路特性完全等效）
y = alpha * y_prev + (1 - alpha) * u;

% 更新状态，为下一个仿真步准备
y_prev = y;

end

== matlab function offGrid_Inverter/rc滤波3 ==
  data: u input; y output
function y = fcn(u)
% 一阶RC低通滤波（数字等效实现）
% 适配：仿真步长 Ts=1e-6s（Fs=1MHz），截止频率 fc=4.7kHz
% 输入：u - 原始信号
% 输出：y - RC滤波后的信号

% persistent 变量保存上一时刻的输出（RC滤波的状态）
persistent y_prev;

% ---------------- 固定参数（已按你的需求预计算） ----------------
fc = 4700;   % 截止频率：4.7kHz
Ts = 1e-6;   % 仿真步长：1us（1e-6s）
tau = 1/(2*pi*fc); % RC时间常数 τ=RC=1/(2πfc)
alpha = exp(-Ts/tau); % 滤波系数（RC离散化核心）
% ----------------------------------------------------------------

% 初始化状态（仅第一次调用时执行，默认初始输出为0）
if isempty(y_prev)
    y_prev = 0;
end

% 一阶RC低通的离散差分方程（和真实RC电路特性完全等效）
y = alpha * y_prev + (1 - alpha) * u;

% 更新状态，为下一个仿真步准备
y_prev = y;

end

== matlab function offGrid_Inverter/滑动平均滤波 ==
  data: IGm_total input; IGm_clean output
function IGm_clean = Notch_100Hz_IGm(IGm_total)
    % 【动态窗口滑动平均滤波】专门消除100Hz纹波
    % 采样频率：20kHz，窗口长度：200点（20kHz/100Hz=200）
    % 核心改进：启动前200个点使用动态窗口，完全消除零值误差
    % 输入：IGm_total - 原始带纹波的电流信号
    % 输出：IGm_clean - 滤波后的平滑电流信号
    
    % 持久变量：仅在第一次调用时初始化，后续调用保留值
    persistent buffer   % 环形数据缓冲区
    persistent index    % 缓冲区当前写入索引
    persistent sum_buf  % 窗口内数据累加和（优化计算，避免循环求和）
    persistent sample_count % 已采样总点数（用于动态窗口判断）
    
    N = 200; % 固定窗口长度：100Hz纹波的精确零点
    
    % ====================== 初始化（仅第一次运行执行） ======================
    if isempty(buffer)
        buffer = zeros(1, N);  % 初始化环形缓冲区为全0
        index = 0;             % 索引从0开始
        sum_buf = 0;           % 累加和初始化为0
        sample_count = 0;      % 采样计数初始化为0
    end
    
    % ====================== 更新索引和计数 ======================
    sample_count = sample_count + 1; % 总采样数+1
    index = index + 1;
    if index > N
        index = 1; % 索引越界时回到起点，实现环形结构
    end
    
    % ====================== 核心滤波逻辑 ======================
    if sample_count <= N
        % ---------------------- 阶段1：动态窗口（前200个点） ----------------------
        % 不除以固定的200，而是除以当前已采样的点数
        % 第1个点：输出 = 第1个点 / 1
        % 第10个点：输出 = 前10个点和 / 10
        % ...
        % 第200个点：输出 = 前200个点和 / 200
        sum_buf = sum_buf + IGm_total;
        buffer(index) = IGm_total;
        IGm_clean = sum_buf / sample_count;
    else
        % ---------------------- 阶段2：标准滑动平均（200个点之后） ----------------------
        % 窗口已满，进入标准滑动模式
        % 减去最旧的采样值，加上最新的采样值
        sum_buf = sum_buf - buffer(index) + IGm_total;
        buffer(index) = IGm_total;
        IGm_clean = sum_buf / N;
    end
end

% 
% function IGm_clean = Notch_100Hz_IGm(IGm_total)
%     % 【标准固定窗口滑动平均滤波】专门消除100Hz纹波
%     % 采样频率：20kHz，窗口长度：200点（20kHz/100Hz=200）
%     % 输入：IGm_total - 原始带纹波的电流信号
%     % 输出：IGm_clean - 滤波后的平滑电流信号
%     
%     % 持久变量：仅在第一次调用时初始化，后续调用保留值
%     persistent buffer   % 环形数据缓冲区
%     persistent index    % 缓冲区当前写入索引
%     persistent sum_buf  % 窗口内数据累加和（优化计算，避免循环求和）
%     
%     N = 200; % 固定窗口长度：100Hz纹波的精确零点
%     
%     % ====================== 初始化（仅第一次运行执行） ======================
%     if isempty(buffer)
%         buffer = zeros(1, N);  % 初始化环形缓冲区为全0
%         index = 0;             % 索引从0开始
%         sum_buf = 0;           % 累加和初始化为0
%     end
%     
%     % ====================== 更新环形缓冲区索引 ======================
%     index = index + 1;
%     if index > N
%         index = 1; % 索引越界时回到起点，实现环形结构
%     end
%     
%     % ====================== 核心滤波逻辑（固定窗口） ======================
%     % 减去最旧的采样值，加上最新的采样值
%     sum_buf = sum_buf - buffer(index) + IGm_total;
%     
%     % 将最新的采样值存入缓冲区
%     buffer(index) = IGm_total;
%     
%     % 计算平均值（滤波输出）
%     IGm_clean = sum_buf / N;
% end

== matlab function offGrid_Inverter/MATLAB Function10 ==
  data: I_ref input; duty_out output; I_fb input
function duty_out = fcn(I_ref, I_fb)
%#codegen
% 同步Boost电流环PI控制器（带钳位抗饱和）
% 适配：20kHz采样、±5A电流传感器、占空比0.1~0.9安全范围
% 输入：
%   I_ref: 电压环输出的电流给定（对应你模型里电压环PI的输出）
%   I_fb: 电流反馈（对应你模型里经过-1增益后的IL信号）
% 输出：
%   duty_out: 最终占空比，直接接你模型里的1/z延迟模块

% 持久化变量：保存积分器状态，每个控制周期保留数值
persistent integral_val;
% 初始化：仅仿真启动的第一个控制周期执行1次
if isempty(integral_val)
    integral_val = 0;
end

% ==================== 1. 控制参数（和你原PI模块参数完全一致，可直接修改）====================
Kp = 0.5;       % 比例增益，和你原设置一致
Ki = 10;         % 积分增益，和你原设置一致
Ts = 5e-5;       % 20kHz控制周期，固定不变
% ==================== 2. 物理极限设置（核心抗饱和阈值）====================
DUTY_MAX = 100;  % 占空比上限，避免上下管直通
DUTY_MIN = -100;  % 占空比下限，杜绝轻载反向电流
I_SAT_LIMIT = 60; % 电流传感器饱和阈值，接近±5A量程提前触发保护

% ==================== 3. 误差计算 ====================
err = I_ref - I_fb;

% ==================== 4. 比例项输出 ====================
prop_out = Kp * err;

% ==================== 5. 核心抗饱和逻辑 ====================
% 5.1 积分项预计算
integral_inc = Ki * Ts * err;
integral_pre = integral_val + integral_inc;
% 5.2 预计算不饱和的PI输出
duty_pre = prop_out + integral_pre;

% 5.3 钳位抗饱和规则：
% 仅当输出在线性区、且电流未达到传感器饱和阈值时，才允许积分累加
% 同时加入反向积分放行规则，避免积分锁死
is_duty_linear = (duty_pre < DUTY_MAX) && (duty_pre > DUTY_MIN);
is_current_unsat = (abs(I_fb) < I_SAT_LIMIT);
is_integral_allow = is_duty_linear && is_current_unsat;
is_reverse_integral = (err > 0 && integral_pre < 0) || (err < 0 && integral_pre > 0);

if is_integral_allow || is_reverse_integral
    integral_val = integral_pre;
end

% ==================== 6. 最终占空比计算 + 硬限幅兜底 ====================
duty_out = prop_out + integral_val;
duty_out = min(max(duty_out, DUTY_MIN), DUTY_MAX);

== matlab function offGrid_Inverter/gemini简便运算版本 ==
  data: u_in input; u_out output
function u_out = RC_CIRCULAR_VALID(u_in)
    persistent buffer ptr;
    % 参数定义 (保持一致)
    N = 400; p = 3; k_rc = 0.3;
    Q0 = 0.25; Q1 = 0.5; Q2 = 0.25;
    
    % 状态变量长度 L = max_order = 402
    L = 402;
    if isempty(buffer)
        buffer = zeros(L, 1);
        ptr = 0; % C语言风格 0 索引
    end

    % --- 1. 计算输出 (对应原代码 b(398)*x(397) + ... ) ---
    % 偏移量计算：原代码 x(n) 对应环形缓冲区的 (ptr + n - 1) % L
    idx397 = mod(ptr + 396, L) + 1;
    idx398 = mod(ptr + 397, L) + 1;
    idx399 = mod(ptr + 398, L) + 1;
    
    % 计算 u_out (k_rc 已包含在 b 中)
    u_out = (k_rc*Q0)*buffer(idx397) + (k_rc*Q1)*buffer(idx398) + (k_rc*Q2)*buffer(idx399);

    % --- 2. 状态更新 (模拟 x(n) = x(n+1) + b*u_in - a*u_out) ---
    % 只有非零系数的位置需要更新
    % 原代码 a(401)=-Q0, 所以 -a(401)*u_out = +Q0*u_out
    buffer(idx397) = buffer(idx397) + (k_rc*Q0)*u_in;
    buffer(idx398) = buffer(idx398) + (k_rc*Q1)*u_in;
    buffer(idx399) = buffer(idx399) + (k_rc*Q2)*u_in;
    
    % 反馈项更新
    idx400 = mod(ptr + 399, L) + 1;
    idx401 = mod(ptr + 400, L) + 1;
    buffer(idx400) = buffer(idx400) + Q0*u_out;
    buffer(idx401) = buffer(idx401) + Q1*u_out;
    
    % 最后一个元素 x(402) 的更新逻辑 (它没有 x(n+1) 可以拉取)
    % 它在当前步被存入，在下一时刻会变成 x(401)
    buffer(ptr + 1) = Q2*u_out;

    % --- 3. 指针移动 ---
    ptr = mod(ptr + 1, L);
end

== matlab function offGrid_Inverter/gemini简便运算版本1，更快捷 ==
  data: u_in input; u_out output
function u_out = RC_VERIFY_INDUSTRIAL(u_in)
    persistent buffer ptr;
    
    % --- 固定参数 (与原代码完全一致) ---
    L = 402;            % 状态数组长度 (max_order)
    k_rc = 0.3;
    Q0 = 0.25; Q1 = 0.5; Q2 = 0.25;
    
    % --- 初始化 ---
    if isempty(buffer)
        buffer = zeros(L, 1);
        ptr = 0;        % 模拟 C 语言的 0 索引
    end

    % --- 1. 工业级索引计算优化 (对应 C 中的 if 判断代替 mod) ---
    % 模拟 C 中的 t397 = p + 396; if(t397 >= L) t397 -= L;
    t397 = ptr + 396; if t397 >= L, t397 = t397 - L; end
    t398 = ptr + 397; if t398 >= L, t398 = t398 - L; end
    t399 = ptr + 398; if t399 >= L, t399 = t399 - L; end
    t400 = ptr + 399; if t400 >= L, t400 = t400 - L; end
    t401 = ptr + 400; if t401 >= L, t401 = t401 - L; end
    
    % MATLAB 访问数组需要 1-based 索引，所以全部 +1
    idx397 = t397 + 1; idx398 = t398 + 1; idx399 = t399 + 1;
    idx400 = t400 + 1; idx401 = t401 + 1;
    idx_ptr = ptr + 1;

    % --- 2. 计算输出 (等效于原代码 u_out = b * x) ---
    u_out = (k_rc * Q0) * buffer(idx397) ...
          + (k_rc * Q1) * buffer(idx398) ...
          + (k_rc * Q2) * buffer(idx399);

    % --- 3. 非规格化数值保护 (工业级截断) ---
    if abs(u_out) < 1e-9, u_out = 0; end

    % --- 4. 增量更新缓冲区 (等效于原代码的 x(n)=x(n+1)+...) ---
    b_u_in = k_rc * u_in;
    buffer(idx397) = buffer(idx397) + Q0 * b_u_in;
    buffer(idx398) = buffer(idx398) + Q1 * b_u_in;
    buffer(idx399) = buffer(idx399) + Q2 * b_u_in;

    buffer(idx400) = buffer(idx400) + Q0 * u_out;
    buffer(idx401) = buffer(idx401) + Q1 * u_out;
    buffer(idx_ptr) = Q2 * u_out; % 对应 x(end) 的赋值

    % --- 5. 指针前进 ---
    ptr = ptr + 1;
    if ptr >= L, ptr = 0; end
end

== matlab function offGrid_Inverter/rc滤波 ==
  data: u input; y output
function y = fcn(u)
% 一阶RC低通滤波（数字等效实现）
% 适配：仿真步长 Ts=1e-6s（Fs=1MHz），截止频率 fc=4.7kHz
% 输入：u - 原始信号
% 输出：y - RC滤波后的信号

% persistent 变量保存上一时刻的输出（RC滤波的状态）
persistent y_prev;

% ---------------- 固定参数（已按你的需求预计算） ----------------
fc = 4700;   % 截止频率：4.7kHz
Ts = 1e-6;   % 仿真步长：1us（1e-6s）
tau = 1/(2*pi*fc); % RC时间常数 τ=RC=1/(2πfc)
alpha = exp(-Ts/tau); % 滤波系数（RC离散化核心）
% ----------------------------------------------------------------

% 初始化状态（仅第一次调用时执行，默认初始输出为0）
if isempty(y_prev)
    y_prev = 0;
end

% 一阶RC低通的离散差分方程（和真实RC电路特性完全等效）
y = alpha * y_prev + (1 - alpha) * u;

% 更新状态，为下一个仿真步准备
y_prev = y;

end

== matlab function offGrid_Inverter/MATLAB Function ==
  data: I_ref input; duty_out output; I_fb input
function duty_out = fcn(I_ref, I_fb)
%#codegen
% 同步Boost电流环PI控制器（带钳位抗饱和）
% 适配：20kHz采样、±5A电流传感器、占空比0.1~0.9安全范围
% 输入：
%   I_ref: 电压环输出的电流给定（对应你模型里电压环PI的输出）
%   I_fb: 电流反馈（对应你模型里经过-1增益后的IL信号）
% 输出：
%   duty_out: 最终占空比，直接接你模型里的1/z延迟模块

% 持久化变量：保存积分器状态，每个控制周期保留数值
persistent integral_val;
% 初始化：仅仿真启动的第一个控制周期执行1次
if isempty(integral_val)
    integral_val = 0;
end

% ==================== 1. 控制参数（和你原PI模块参数完全一致，可直接修改）====================
Kp = 0.05;       % 比例增益，和你原设置一致
Ki = 10;         % 积分增益，和你原设置一致
Ts = 5e-5;       % 20kHz控制周期，固定不变
% ==================== 2. 物理极限设置（核心抗饱和阈值）====================
DUTY_MAX = 0.9;  % 占空比上限，避免上下管直通
DUTY_MIN = 0.1;  % 占空比下限，杜绝轻载反向电流
I_SAT_LIMIT = 5.0; % 电流传感器饱和阈值，接近±5A量程提前触发保护

% ==================== 3. 误差计算 ====================
err = I_ref - I_fb;

% ==================== 4. 比例项输出 ====================
prop_out = Kp * err;

% ==================== 5. 核心抗饱和逻辑 ====================
% 5.1 积分项预计算
integral_inc = Ki * Ts * err;
integral_pre = integral_val + integral_inc;
% 5.2 预计算不饱和的PI输出
duty_pre = prop_out + integral_pre;

% 5.3 钳位抗饱和规则：
% 仅当输出在线性区、且电流未达到传感器饱和阈值时，才允许积分累加
% 同时加入反向积分放行规则，避免积分锁死
is_duty_linear = (duty_pre < DUTY_MAX) && (duty_pre > DUTY_MIN);
is_current_unsat = (abs(I_fb) < I_SAT_LIMIT);
is_integral_allow = is_duty_linear && is_current_unsat;
is_reverse_integral = (err > 0 && integral_pre < 0) || (err < 0 && integral_pre > 0);

if is_integral_allow || is_reverse_integral
    integral_val = integral_pre;
end

% ==================== 6. 最终占空比计算 + 硬限幅兜底 ====================
duty_out = prop_out + integral_val;
duty_out = min(max(duty_out, DUTY_MIN), DUTY_MAX);

== matlab function offGrid_Inverter/MATLAB Function2 ==
  data: t input; y output
function y = smooth_rise(t)
% 功能：输入时间t，输出0.3秒内从0平滑曲线增长到32
% 曲线类型：余弦缓升（无超调、无冲击，工业控制标准）
% 规则：
%   t < 0        → 输出 0
%   0 ≤ t ≤ 0.3s → 平滑从 0 增长到 32
%   t > 0.3s     → 保持 32

T = 0.3;   % 总上升时间 0.3秒
A = 55;    % 目标值

if t < 0
    y = 0;
elseif t <= T
    % 余弦平滑增长公式
    tau = t / T;
    smooth_curve = 0.5 * (1 - cos(pi * tau));
    y = A * smooth_curve;
else
    y = A;
end
end

== matlab function offGrid_Inverter/MATLAB Function3 ==
  data: I_ref input; duty_out output; I_fb input
function duty_out = fcn(I_ref, I_fb)
%#codegen
% 同步Boost电流环PI控制器（带钳位抗饱和）
% 适配：20kHz采样、±5A电流传感器、占空比0.1~0.9安全范围
% 输入：
%   I_ref: 电压环输出的电流给定（对应你模型里电压环PI的输出）
%   I_fb: 电流反馈（对应你模型里经过-1增益后的IL信号）
% 输出：
%   duty_out: 最终占空比，直接接你模型里的1/z延迟模块

% 持久化变量：保存积分器状态，每个控制周期保留数值
persistent integral_val;
% 初始化：仅仿真启动的第一个控制周期执行1次
if isempty(integral_val)
    integral_val = 0;
end

% ==================== 1. 控制参数（和你原PI模块参数完全一致，可直接修改）====================
Kp = 0.05;       % 比例增益，和你原设置一致
Ki = 4000;         % 积分增益，和你原设置一致
Ts = 5e-5;       % 20kHz控制周期，固定不变
% ==================== 2. 物理极限设置（核心抗饱和阈值）====================
DUTY_MAX = 1000;  % 占空比上限，避免上下管直通
DUTY_MIN = -1000;  % 占空比下限，杜绝轻载反向电流
I_SAT_LIMIT = 50.0; % 电流传感器饱和阈值，接近±5A量程提前触发保护

% ==================== 3. 误差计算 ====================
err = I_ref - I_fb;

% ==================== 4. 比例项输出 ====================
prop_out = Kp * err;

% ==================== 5. 核心抗饱和逻辑 ====================
% 5.1 积分项预计算
integral_inc = Ki * Ts * err;
integral_pre = integral_val + integral_inc;
% 5.2 预计算不饱和的PI输出
duty_pre = prop_out + integral_pre;

% 5.3 钳位抗饱和规则：
% 仅当输出在线性区、且电流未达到传感器饱和阈值时，才允许积分累加
% 同时加入反向积分放行规则，避免积分锁死
is_duty_linear = (duty_pre < DUTY_MAX) && (duty_pre > DUTY_MIN);
is_current_unsat = (abs(I_fb) < I_SAT_LIMIT);
is_integral_allow = is_duty_linear && is_current_unsat;
is_reverse_integral = (err > 0 && integral_pre < 0) || (err < 0 && integral_pre > 0);

if is_integral_allow || is_reverse_integral
    integral_val = integral_pre;
end

% ==================== 6. 最终占空比计算 + 硬限幅兜底 ====================
duty_out = prop_out + integral_val;
duty_out = min(max(duty_out, DUTY_MIN), DUTY_MAX);

== matlab function offGrid_Inverter/MATLAB Function4 ==
  data: I_ref input; duty_out output; I_fb input
function duty_out = fcn(I_ref, I_fb)
%#codegen
% 同步Boost电流环PI控制器（带钳位抗饱和）
% 适配：20kHz采样、±5A电流传感器、占空比0.1~0.9安全范围
% 输入：
%   I_ref: 电压环输出的电流给定（对应你模型里电压环PI的输出）
%   I_fb: 电流反馈（对应你模型里经过-1增益后的IL信号）
% 输出：
%   duty_out: 最终占空比，直接接你模型里的1/z延迟模块

% 持久化变量：保存积分器状态，每个控制周期保留数值
persistent integral_val;
% 初始化：仅仿真启动的第一个控制周期执行1次
if isempty(integral_val)
    integral_val = 0;
end

% ==================== 1. 控制参数（和你原PI模块参数完全一致，可直接修改）====================
Kp = 0.1;       % 比例增益，和你原设置一致
Ki = 0;         % 积分增益，和你原设置一致
Ts = 5e-5;       % 20kHz控制周期，固定不变
% ==================== 2. 物理极限设置（核心抗饱和阈值）====================
DUTY_MAX = 0.9;  % 占空比上限，避免上下管直通
DUTY_MIN = -0.9;  % 占空比下限，杜绝轻载反向电流
I_SAT_LIMIT = 10.0; % 电流传感器饱和阈值，接近±5A量程提前触发保护

% ==================== 3. 误差计算 ====================
err = I_ref - I_fb;

% ==================== 4. 比例项输出 ====================
prop_out = Kp * err;

% ==================== 5. 核心抗饱和逻辑 ====================
% 5.1 积分项预计算
integral_inc = Ki * Ts * err;
integral_pre = integral_val + integral_inc;
% 5.2 预计算不饱和的PI输出
duty_pre = prop_out + integral_pre;

% 5.3 钳位抗饱和规则：
% 仅当输出在线性区、且电流未达到传感器饱和阈值时，才允许积分累加
% 同时加入反向积分放行规则，避免积分锁死
is_duty_linear = (duty_pre < DUTY_MAX) && (duty_pre > DUTY_MIN);
is_current_unsat = (abs(I_fb) < I_SAT_LIMIT);
is_integral_allow = is_duty_linear && is_current_unsat;
is_reverse_integral = (err > 0 && integral_pre < 0) || (err < 0 && integral_pre > 0);

if is_integral_allow || is_reverse_integral
    integral_val = integral_pre;
end

% ==================== 6. 最终占空比计算 + 硬限幅兜底 ====================
duty_out = prop_out + integral_val;
duty_out = min(max(duty_out, DUTY_MIN), DUTY_MAX);
